simulink model "IEEE9_16b_1"  (R2020a)
settings: Solver=ode15s  StartTime=0.0  StopTime=5  MaxStep=1e-4  RelTol=1e-3
undefined symbols (not defined in the file or in its folder): k
libraries: powerlib_meascontrol x29, powerlib x27, simulink_extras x26, sps_avr x3
(part 1 of 2)
settings Model: Creator=Pankaj  LastModifiedBy=ahmed
settings DataIOCC: ReturnWorkspaceOutputs=off
settings DebuggingCC: UnconnectedInputMsg=none  UnconnectedOutputMsg=none  UnconnectedLineMsg=none  ArithmeticOperatorsInVariantConditions=warning
settings SFSimCC: SimUseLocalCustomCode=off  CustomCodeUndefinedFunction=UseInterfaceOnly
settings RTWCC: RTWUseLocalCustomCode=off
settings CodeAppCC: StateflowObjectComments=on
settings SimscapeCC: SimscapeNormalizeSystem=off

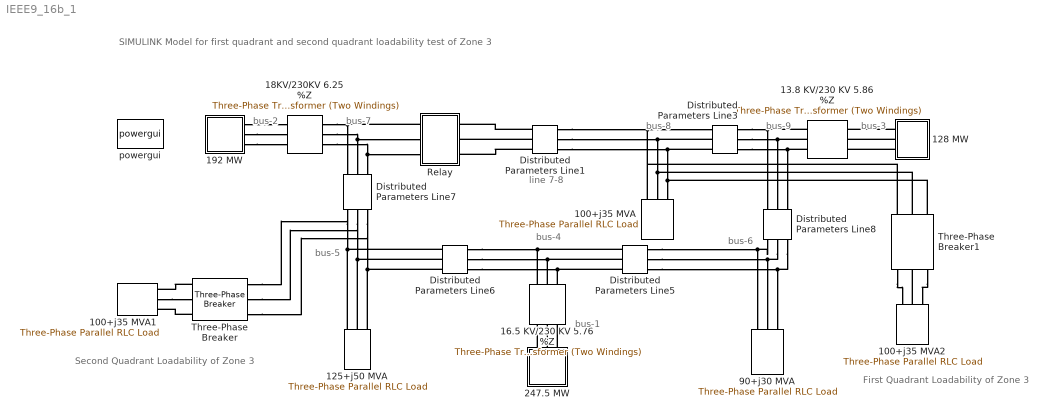
== system IEEE9_16b_1 ==
  note: Second Quadrant Loadability of Zone 3
  note: SIMULINK Model for first quadrant and second quadrant loadability test of Zone 3
  note: bus-2
  note: bus-7
  note: bus-8
  note: bus-9
  note: bus-1
  note: bus-3
  note: bus-4
  note: bus-6
  note: bus-5
  note: line 7-8
  note: First Quadrant Loadability of Zone 3
  100+j35 MVA : powerlib/Elements/Three-Phase Parallel RLC Load  LConnTagsString=A|B|C  Configuration=Y (grounded)  NominalVoltage=(230000)*0.993698  Vabc=[1e3 1e3 1e3]  Vabcp=[1e3 1e3 1e3]  NominalFrequency=60  UnbalancedPower=off  ActivePower=100e6  InductivePower=35e6  CapacitivePower=0  Pabc=[10e3 9e3 11e3]  QLabc=[100 90 110]  QCabc=[100 90 110]  Pabcp=[10e3 9e3 11e3]  QLabcp=[100 90 110]  QCabcp=[100 90 110]  Measurements=None  LoadType=constant PQ
  100+j35 MVA1 : powerlib/Elements/Three-Phase Parallel RLC Load  LConnTagsString=A|B|C  Configuration=Y (grounded)  NominalVoltage=(230000)*0.993698  Vabc=[1e3 1e3 1e3]  Vabcp=[1e3 1e3 1e3]  NominalFrequency=60  UnbalancedPower=off  ActivePower=1.7469e+15  InductivePower=1.0085e+15  CapacitivePower=0  Pabc=[10e3 9e3 11e3]  QLabc=[100 90 110]  QCabc=[100 90 110]  Pabcp=[10e3 9e3 11e3]  QLabcp=[100 90 110]  QCabcp=[100 90 110]  Measurements=None  LoadType=constant PQ
  100+j35 MVA2 : powerlib/Elements/Three-Phase Parallel RLC Load  LConnTagsString=A|B|C  Configuration=Y (grounded)  NominalVoltage=(230000)*0.993698  Vabc=[1e3 1e3 1e3]  Vabcp=[1e3 1e3 1e3]  NominalFrequency=60  UnbalancedPower=off  ActivePower=1.7469e+15  InductivePower=1.0085e+15  CapacitivePower=0  Pabc=[10e3 9e3 11e3]  QLabc=[100 90 110]  QCabc=[100 90 110]  Pabcp=[10e3 9e3 11e3]  QLabcp=[100 90 110]  QCabcp=[100 90 110]  Measurements=None  LoadType=constant PQ
  125+j50 MVA : powerlib/Elements/Three-Phase Parallel RLC Load  LConnTagsString=A|B|C  Configuration=Y (grounded)  NominalVoltage=(223027)*1  Vabc=[1e3 1e3 1e3]  Vabcp=[1e3 1e3 1e3]  NominalFrequency=60  UnbalancedPower=off  ActivePower=125e6  InductivePower=50e6  CapacitivePower=0  Pabc=[10e3 9e3 11e3]  QLabc=[100 90 110]  QCabc=[100 90 110]  Pabcp=[10e3 9e3 11e3]  QLabcp=[100 90 110]  QCabcp=[100 90 110]  Measurements=None  LoadType=constant PQ
  128 MW : Subsystem
  13.8 KV/230 KV 5.86 %Z : powerlib/Elements/Three-Phase Transformer (Two Windings)  Winding1Connection=Yg  Winding2Connection=Yg  CoreType=Three single-phase transformers  SetSaturation=off  Hysteresis=off  DataFile='hysteresis'  SetInitialFlux=off  Measurements=None  UNITS=pu  NominalPower=[ 100e6 , 60 ]  Winding1=[13.8e3 , 1e-6 , 0 ]  Winding2=[ 230e3 , 1e-6, 0.0586 ]  Rm=500  Lm=500  L0=0.5  Saturation=[ 0,0 ; 0.0024,1.2 ; 1.0,1.52 ]  InitialFluxes=[ 0.8 , -0.8 , 0.7 ]  BreakLoop=off  DiscreteSolver=Trapezoidal iterative  DataType=off  TransfoNumber=1
  "16.5 KV/230 KV 5.76 %Z     " : powerlib/Elements/Three-Phase Transformer (Two Windings)  Winding1Connection=Yg  Winding2Connection=Yg  CoreType=Three single-phase transformers  SetSaturation=off  Hysteresis=off  DataFile='hysteresis'  SetInitialFlux=off  Measurements=None  UNITS=pu  NominalPower=[ 100e6 , 60 ]  Winding1=[16.5e3 , 1e-6, 0 ]  Winding2=[ 230e3 ,1e-6, 0.0576 ]  Rm=500  Lm=500  L0=0.5  Saturation=[ 0,0 ; 0.0024,1.2 ; 1.0,1.52 ]  InitialFluxes=[ 0.8 , -0.8 , 0.7 ]  BreakLoop=off  DiscreteSolver=Trapezoidal iterative  DataType=off  TransfoNumber=1
  18KV/230KV 6.25 %Z : powerlib/Elements/Three-Phase Transformer (Two Windings)  Winding1Connection=Yg  Winding2Connection=Yg  CoreType=Three single-phase transformers  SetSaturation=off  Hysteresis=off  DataFile='hysteresis'  SetInitialFlux=off  Measurements=None  UNITS=pu  NominalPower=[ 100e6 , 60 ]  Winding1=[ 18e3 , 1e-6 , 0]  Winding2=[ 230e3 , 1e-6, 0.0625 ]  Rm=500  Lm=500  L0=0.5  Saturation=[ 0,0 ; 0.0024,1.2 ; 1.0,1.52 ]  InitialFluxes=[ 0.8 , -0.8 , 0.7 ]  BreakLoop=off  DiscreteSolver=Trapezoidal iterative  DataType=off  TransfoNumber=1
  192 MW : Subsystem
  247.5 MW : Subsystem
  90+j30 MVA : powerlib/Elements/Three-Phase Parallel RLC Load  LConnTagsString=A|B|C  Configuration=Y (grounded)  NominalVoltage=(226177)*0.999999  Vabc=[1e3 1e3 1e3]  Vabcp=[1e3 1e3 1e3]  NominalFrequency=60  UnbalancedPower=off  ActivePower=90e6  InductivePower=30e6  CapacitivePower=0  Pabc=[10e3 9e3 11e3]  QLabc=[100 90 110]  QCabc=[100 90 110]  Pabcp=[10e3 9e3 11e3]  QLabcp=[100 90 110]  QCabcp=[100 90 110]  Measurements=None  LoadType=constant PQ
  Distributed Parameters Line1 : powerlib/Elements/Distributed Parameters Line  Phases=3  Frequency=60  Resistance=[0.044965 0.11241]  Inductance="[1.01e-3  2.02e-3]"  Capacitance=[12.74e-9 7.751e-9]  Length=100  x1=[-0.0004 1.93656449270455e-06 23508.2160177902 -52538.75935175;-0.00035 1.67378461087068e-06 24494.3184666325 -52086.3350065214;-0.0003 1.4104100413345e-06 25471.7182007562 -51615.4046344802;-0.00025 1.14653435982647e-06 26440.0679546897 -51126.1355549453;-0.0002 8.82251320119748e-07 27399.0236783764 -50618.7016028908;-0.00015 6.17654820719931e-07 28348.2446594139 -50093.2830671837;-0.0001 3.52838871503349e-07 29287.3936441074 -49550.0666265279;-5e-05 8.78975603158065e-08 30216.1369572946 -48989.2452831382]  x2=[-0.0004 4.18624145948892e-06 28259.244689254 -52398.8670670216;-0.00035 3.9633430905482e-06 29241.8663646278 -51856.9185470287;-0.0003 3.73903656467934e-06 30214.0985441207 -51296.5455107989;-0.00025 3.51340157692291e-06 31175.595798269 -50717.9470562037;-0.0002 3.28651829431568e-06 32126.0165116764 -50121.3287565189;-0.00015 3.05846732740762e-06 33065.023004389 -49506.9025873855;-0.0001 2.82932970162139e-06 33992.2816518711 -48874.8868514958;-5e-05 2.59918682846436e-06 34907.4630035407 -48225.5061010312]  x3=[-0.0004 -1.73044531826081e-08 87.9731080176391 -312.019576771818;-0.00035 -1.71851910893741e-08 93.8385916181453 -310.305999768085;-0.0003 -1.70598231795753e-08 99.6707348138731 -308.482172520194;-0.00025 -1.69283939958332e-08 105.467465472116 -306.54874302528;-0.0002 -1.67909502343109e-08 111.226724042071 -304.506398221637;-0.00015 -1.66475407281225e-08 116.946464286594 -302.355863744649;-0.0001 -1.64982164299825e-08 122.624654009211 -300.097903668976;-5e-05 -1.63430303941032e-08 128.259275776149 -297.733320237081]  x4=[-0.0004 3.28235405138543e-08 68.6553647797155 -68.5872480221798;-0.00035 3.17845507984995e-08 69.935937439127 -67.2810236786274;-0.0003 3.07342681835919e-08 71.1916621929746 -65.9508947077285;-0.00025 2.96730658295436e-08 72.4220928882326 -64.5973336979729;-0.0002 2.86013207764978e-08 73.6267923587337 -63.2208215631423;-0.00015 2.75194138103686e-08 74.8053325804924 -61.8218473714436;-0.0001 2.64277293275496e-08 75.9572948237797 -60.400908171746;-5e-05 2.53266551983393e-08 77.0822698018957 -58.9585088169809]  x5=0.000395689524753941  V1=ones(3,3)  V2=ones(3,3)  I1=ones(3,3)  I2=ones(3,3)  nHarmo=1  Measurements=None
  Distributed Parameters Line3 : powerlib/Elements/Distributed Parameters Line  Phases=3  Frequency=60  Resistance=[ 0.062951 0.15737]  Inductance="[ 1.414e-3  3.53e-3]"  Capacitance=[12.74e-9 7.751e-9]  Length=100  x1=[-0.00055 4.84569834764548e-06 0 0;-0.0005 4.62749747611836e-06 0 0;-0.00045 4.40765247677236e-06 27266.5826388019 -52922.198519049;-0.0004 4.18624145948892e-06 28259.244689254 -52398.8670670216;-0.00035 3.9633430905482e-06 29241.8663646278 -51856.9185470287;-0.0003 3.73903656467934e-06 30214.0985441207 -51296.5455107989;-0.00025 3.51340157692291e-06 31175.595798269 -50717.9470562037;-0.0002 3.28651829431568e-06 32126.0165116764 -50121.3287565189;-0.00015 3.05846732740762e-06 33065.023004389 -49506.9025873855;-0.0001 2.82932970162139e-06 33992.2816518711 -48874.8868514958;-5e-05 2.59918682846436e-06 34907.4630035407 -48225.5061010312]  x2=[-0.00055 6.18158400270898e-06 0 0;-0.0005 5.99518973223753e-06 0 0;-0.00045 5.80666539940102e-06 39827.4813836401 -51273.9727441437;-0.0004 5.61607798599722e-06 40786.8453796834 -50514.1819455975;-0.00035 5.42349520682662e-06 41731.7180037748 -49736.4436987352;-0.0003 5.22898548563364e-06 42661.7635471699 -48941.0343302528;-0.00025 5.03261793079605e-06 43576.6515691157 -48128.2364453113;-0.0002 4.83446231077106e-06 44476.0570142543 -47298.338827129;-0.00015 4.63458902930691e-06 45359.6603281138 -46451.6363343782;-0.0001 4.43306910042879e-06 46227.1475706441 -45588.4297964226;-5e-05 4.22997412320786e-06 47078.2105277586 -44709.0259064351]  x3=[-0.00055 -2.65416129090466e-09 0 0;-0.0005 -2.74354657868112e-09 0 0;-0.00045 -2.83195709742188e-09 125.571553781947 -390.764061979304;-0.0004 -2.91936143529064e-09 132.914576268336 -388.327827737904;-0.00035 -3.00572853794231e-09 140.210374838665 -385.753622468377;-0.0003 -3.09102771955659e-09 147.456357330443 -383.042360773598;-0.00025 -3.1752286737404e-09 154.649949280592 -380.195005951937;-0.0002 -3.25830148429566e-09 161.788594840145 -377.212569655006;-0.00015 -3.34021663584833e-09 168.869757682328 -374.096111528218;-0.0001 -3.42094502433513e-09 175.890921903699 -370.846738834307;-5e-05 -3.50045796734401e-09 182.849592918043 -367.465606059919]  x4=[-0.00055 2.18052139273402e-08 0 0;-0.0005 2.13350493540652e-08 0 0;-0.00045 2.0857304539344e-08 48.1436321371247 66.4160212313476;-0.0004 2.03721492236346e-08 46.8832348550945 67.3116503579346;-0.00035 1.98797557803104e-08 45.6061801829603 68.1833639756619;-0.0003 1.93802991544172e-08 44.3129218521663 69.0308523688317;-0.00025 1.88739568005161e-08 43.0039193512395 69.8538144288535;-0.0002 1.83609086196343e-08 41.6796377625354 70.6519577612259;-0.00015 1.78413368953475e-08 40.3405475969968 71.4249987894233;-0.0001 1.73154262290155e-08 38.9871246269832 72.1726628556494;-5e-05 1.67833634741938e-08 37.6198497172315 72.8946843184216]  x5=0.000523077718890797  V1=ones(3,3)  V2=ones(3,3)  I1=ones(3,3)  I2=ones(3,3)  nHarmo=1  Measurements=None
  Distributed Parameters Line5 : powerlib/Elements/Distributed Parameters Line  Phases=3  Frequency=60  Resistance=[ 0.08993 0.224825]  Inductance="[ 1.29e-3  3.22e-3]"  Capacitance=[12.74e-9 7.751e-9]  Length=100  x1=[-0.0005 7.68678845069513e-06 29544.2185806977 -56120.4339666881;-0.00045 7.56630098616658e-06 30596.7580663869 -55553.6046883368;-0.0004 7.44312525092549e-06 31638.4266696252 -54967.0374787648;-0.00035 7.31730500872407e-06 32668.8542905178 -54360.9407425086;-0.0003 7.18888496289525e-06 33687.6748230377 -53735.5298228527;-0.00025 7.05791074046985e-06 34694.5262851008 -53091.0269253187;-0.0002 6.92442887596542e-06 35689.0509471768 -52427.6610387174;-0.00015 6.78848679485286e-06 36670.895459389 -51745.6678537895;-0.0001 6.65013279670626e-06 37639.7109770572 -51045.2896794663;-5e-05 6.50941603804239e-06 38595.1532846412 -50326.7753567781]  x2=[-0.0005 7.53028054430953e-06 29320.5644209634 -55402.7114798878;-0.00045 7.41145500534729e-06 30359.6156210989 -54840.2252139311;-0.0004 7.28999621171217e-06 31387.8801943652 -54258.254477084;-0.00035 7.1659473171352e-06 32404.9928032554 -53657.0060407782;-0.0003 7.03935239559796e-06 33410.5920725029 -53036.6935257204;-0.00025 6.91025642567326e-06 34404.3207174755 -52397.5373259933;-0.0002 6.77870527454453e-06 35385.8256711174 -51739.7645307514;-0.00015 6.64474568170936e-06 36354.7582093921 -51063.6088435367;-0.0001 6.50842524237322e-06 37310.7740751826 -50369.3104992453;-5e-05 6.36979239053909e-06 38253.5336006037 -49657.1161787729]  x3=[-0.0005 1.16182688102649e-08 90.9008008515084 -172.669734952446;-0.00045 1.14361622704147e-08 94.1392240277942 -170.925730953576;-0.0004 1.12499925165645e-08 97.3441999860379 -169.120997856382;-0.00035 1.10598256939413e-08 100.514590013543 -167.256176873939;-0.0003 1.08657293679117e-08 103.649267685827 -165.331930568262;-0.00025 1.06677724999762e-08 106.747119266842 -163.348942614903;-0.0002 1.04660254232673e-08 109.80704410467 -161.307917560037;-0.00015 1.02605598175607e-08 112.827955022586 -159.209580570149;-0.0001 1.00514486838078e-08 115.808778705327 -157.054677174379;-5e-05 9.83876631819869e-09 118.748456080431 -154.843972999644]  x4=[-0.0005 1.31880150263936e-08 63.7477174436907 -184.411908073343;-0.00045 1.30494088536706e-08 67.2122870580504 -183.177608782538;-0.0004 1.29061662881181e-08 70.6529764668576 -181.878227359555;-0.00035 1.27583382231376e-08 74.0685632095486 -180.514225468425;-0.0003 1.26059771813369e-08 77.4578337444175 -179.086087732526;-0.00025 1.24491372958684e-08 80.8195838797816 -177.594321562396;-0.0002 1.22878742911968e-08 84.1526192018252 -176.039456975451;-0.00015 1.21222454632996e-08 87.455755498969 -174.422046407674;-0.0001 1.19523096593109e-08 90.727819182615 -172.742664517341;-5e-05 1.17781272566125e-08 93.9676477041165 -171.001907980839]  x5=0.000499582025297148  V1=ones(3,3)  V2=ones(3,3)  I1=ones(3,3)  I2=ones(3,3)  nHarmo=1  Measurements=None
  Distributed Parameters Line6 : powerlib/Elements/Distributed Parameters Line  Phases=3  Frequency=60  Resistance=[ 0.0529 0.13225]  Inductance="[ 1.192e-3  2.38e-3]"  Capacitance=[12.74e-9 7.751e-9]  Length=100  x1=[-0.00045 -5.95947459759956e-05 0 0;-0.0004 -5.89390235964401e-05 52397.5683409792 -216748.374353491;-0.00035 -5.82623604624459e-05 56473.6196200629 -215722.25524866;-0.0003 -5.75649969892026e-05 60529.6060910015 -214619.491053726;-0.00025 -5.68471809466315e-05 64564.0866811148 -213440.473575556;-0.0002 -5.61091673713546e-05 68575.6279586598 -212185.621713448;-0.00015 -5.53512184760811e-05 72562.804642122 -210855.381310291;-0.0001 -5.45736035564444e-05 76524.2001066113 -209450.224994168;-5e-05 -5.37765988953227e-05 80458.4068871817 -207970.652010426]  x2=[-0.00045 -6.03278555922693e-05 0 0;-0.0004 -5.98632667464564e-05 67525.6481000577 -218721.992470464;-0.00035 -5.93774087670144e-05 71636.2113908087 -217410.381331028;-0.0003 -5.88704542769701e-05 75721.3226767569 -216021.525318331;-0.00025 -5.83425833948398e-05 79779.5305373141 -214555.9178863;-0.0002 -5.77939836706344e-05 83809.393110551 -213014.079758277;-0.00015 -5.72248500192237e-05 87809.478605484 -211396.558742008;-0.0001 -5.66353846510841e-05 91778.3658107837 -209703.929535008;-5e-05 -5.6025797000454e-05 95714.6445997244 -207936.793520373]  x3=[-0.00045 -1.88034187860694e-09 0 0;-0.0004 -1.35212413892515e-09 113.008036792422 -1047.40700837275;-0.00035 -8.23425995975107e-10 132.729903038659 -1045.09091125901;-0.0003 -2.94435293689531e-10 152.404610982357 -1042.40349832082;-0.00025 2.34660020053904e-10 172.025170293465 -1039.3457243832;-0.0002 7.63671960209575e-10 191.584609880685 -1035.91867585868;-0.00015 1.2924125713541e-09 211.075980368268 -1032.12357036127;-0.0001 1.82069399446599e-09 230.492356565089 -1027.96175627389;-5e-05 2.34832853367111e-09 249.826839925139 -1023.43471226927]  x4=[-0.00045 -2.19129648768199e-07 0 0;-0.0004 -2.17997545895897e-07 170.130050868707 -386.485135338421;-0.00035 -2.16787989533558e-07 177.384455284088 -383.209783742097;-0.0003 -2.155014094308e-07 184.575835847143 -379.798279534308;-0.00025 -2.14138262703407e-07 191.701637494601 -376.251834806255;-0.0002 -2.1269903367092e-07 198.759328463067 -372.571709592863;-0.00015 -2.11184233684561e-07 205.746401188547 -368.759211425096;-0.0001 -2.09594400945552e-07 212.66037319737 -364.815694865401;-5e-05 -2.07930100313896e-07 219.498787988203 -360.742561026432]  x5=0.000429504132692574  V1=ones(3,3)  V2=ones(3,3)  I1=ones(3,3)  I2=ones(3,3)  nHarmo=1  Measurements=None
  Distributed Parameters Line7 : powerlib/Elements/Distributed Parameters Line  Phases=3  Frequency=60  Resistance=[ 0.16928 0.4232]  Inductance="[ 2.259e-3  5.64e-3]"  Capacitance=[12.74e-9 7.751e-9]  Length=100  x1=[-0.0007 -2.13875531402635e-06 6576.06110071559 -50761.5133016491;-0.00065 -2.51023483495657e-06 7531.67302268626 -50628.5477731784;-0.0006 -2.88082248140271e-06 8484.60897709492 -50477.5941627577;-0.00055 -3.25038658533858e-06 9434.53039033448 -50308.706103486;-0.0005 -3.61879584239778e-06 10381.09975985 -50121.9436004865;-0.00045 -3.9859193585255e-06 11323.9807740517 -49917.3730095873;-0.0004 -4.35162669648456e-06 12262.8384318048 -49695.0670137453;-0.00035 -4.71578792219914e-06 13197.339161454 -49455.1045972223;-0.0003 -5.07827365091974e-06 14127.1509393399 -49197.5710175221;-0.00025 -5.43895509319298e-06 15051.9434077651 -48922.5577750995;-0.0002 -5.79770410061983e-06 15971.3879923692 -48630.1625808499;-0.00015 -6.15439321138618e-06 16885.1580188692 -48320.4893213936;-0.0001 -6.50889569554939e-06 17792.9288291257 -47993.6480221651;-5e-05 -6.86108560006486e-06 18694.3778964925 -47649.7548083218]  x2=[-0.0007 3.49554589550201e-06 17428.6650067406 -54856.1444386474;-0.00065 3.23828508115508e-06 18459.5267865558 -54517.8978888896;-0.0006 2.97987371953829e-06 19483.8299844009 -54160.2813896054;-0.00055 2.72040362297797e-06 20501.2106702271 -53783.4220002339;-0.0005 2.45996697996393e-06 21511.3073735211 -53387.4536171219;-0.00045 2.19865632239533e-06 22513.761211734 -52972.5169259504;-0.0004 1.93656449270455e-06 23508.2160177902 -52538.75935175;-0.00035 1.67378461087068e-06 24494.3184666325 -52086.3350065214;-0.0003 1.4104100413345e-06 25471.7182007562 -51615.4046344802;-0.00025 1.14653435982647e-06 26440.0679546897 -51126.1355549453;-0.0002 8.82251320119748e-07 27399.0236783764 -50618.7016028908;-0.00015 6.17654820719931e-07 28348.2446594139 -50093.2830671837;-0.0001 3.52838871503349e-07 29287.3936441074 -49550.0666265279;-5e-05 8.78975603158065e-08 30216.1369572946 -48989.2452831382]  x3=[-0.0007 -2.19263741189959e-08 -18.6535496892831 -248.528127503515;-0.00065 -2.17734559243906e-08 -13.9658449001845 -248.835565608354;-0.0006 -2.16128017245723e-08 -9.27317811289293 -249.054593621594;-0.00055 -2.14444685992131e-08 -4.57721660957317 -249.185133723622;-0.0005 -2.1268516356271e-08 0.120371157013008 -249.227139534162;-0.00045 -2.108500751074e-08 4.81791615630025 -249.180596128751;-0.0004 -2.08940072624393e-08 9.51374937291826 -249.045520044038;-0.00035 -2.06955834728475e-08 14.2062023996849 -248.821959271913;-0.0003 -2.04898066409922e-08 18.8936080303834 -248.509993242453;-0.00025 -2.0276749878402e-08 23.5743008521129 -248.109732795705;-0.0002 -2.00564888831302e-08 28.2466178370015 -247.621320142297;-0.00015 -1.98291019128595e-08 32.9088989330721 -247.044928812922;-0.0001 -1.95946697570979e-08 37.5594876540515 -246.380763596672;-5e-05 -1.93532757084738e-08 42.1967316679113 -245.629060468288]  x4=[-0.0007 2.82358103925018e-08 49.0199394768717 -0.498718947797115;-0.00065 2.73756427817605e-08 49.0206313214662 0.425314365616468;-0.0006 2.65057487354913e-08 49.0039063691698 1.34919656686113;-0.00055 2.56264373229066e-08 48.9697705622783 2.27259940498995;-0.0005 2.47380209591643e-08 48.9182360290814 3.19519479937143;-0.00045 2.38408152943683e-08 48.8493210795532 4.11665495625499;-0.0004 2.2935139101419e-08 48.7630501988474 5.03665248523452;-0.00035 2.20213141627554e-08 48.6594540385968 5.95486051556867;-0.0003 2.10996651560268e-08 48.5385694060241 6.87095281231641;-0.00025 2.01705195387369e-08 48.4004392508636 7.78460389224679;-0.0002 1.92342074318991e-08 48.2451126501017 8.69548913948156;-0.00015 1.82910615027468e-08 48.0726447905399 9.60328492082967;-0.0001 1.73414168465375e-08 47.8830969491877 10.5076687007726;-5e-05 1.63856108674959e-08 47.6765364714904 11.4083191560596]  x5=0.000661178039562719  V1=ones(3,3)  V2=ones(3,3)  I1=ones(3,3)  I2=ones(3,3)  nHarmo=1  Measurements=None
  Distributed Parameters Line8 : powerlib/Elements/Distributed Parameters Line  Phases=3  Frequency=60  Resistance=[ 0.20631 0.5157]  Inductance="[ 2.38e-3  6.09e-3]"  Capacitance=[12.74e-9 7.751e-9]  Length=100  x1=[-0.0007 7.97841966236929e-06 25063.9314735538 -57453.9201757617;-0.00065 7.87053977796756e-06 26142.4011326644 -56971.3000027424;-0.0006 7.75986352825922e-06 27211.5825211327 -56468.4381981077;-0.00055 7.6464302359888e-06 28271.0957639024 -55945.5134262624;-0.0005 7.53028020346491e-06 29320.5644209634 -55402.7114798878;-0.00045 7.41145469824105e-06 30359.6156210989 -54840.2252139311;-0.0004 7.28999593845341e-06 31387.8801943652 -54258.254477084;-0.00035 7.16594707782102e-06 32404.9928032554 -53657.0060407782;-0.0003 7.03935219031339e-06 33410.5920725029 -53036.6935257204;-0.00025 6.91025625449124e-06 34404.3207174755 -52397.5373259933;-0.0002 6.77870513752587e-06 35385.8256711174 -51739.7645307514;-0.00015 6.64474557890275e-06 36354.7582093921 -51063.6088435367;-0.0001 6.50842517381518e-06 37310.7740751826 -50369.3104992453;-5e-05 6.36979235625398e-06 38253.5336006037 -49657.1161787729]  x2=[-0.0007 6.72732811486975e-06 34825.3942087243 -54794.4952491998;-0.00065 6.5477182369001e-06 35852.0035042055 -54128.3601017747;-0.0006 6.36578198581861e-06 36865.8747535553 -53442.993405744;-0.00055 6.18158400270898e-06 37866.6477331464 -52738.6386686313;-0.0005 5.99518973223753e-06 38853.9668731044 -52015.546144321;-0.00045 5.80666539940102e-06 39827.4813836401 -51273.9727441437;-0.0004 5.61607798599722e-06 40786.8453796834 -50514.1819455975;-0.00035 5.42349520682662e-06 41731.7180037748 -49736.4436987352;-0.0003 5.22898548563364e-06 42661.7635471699 -48941.0343302528;-0.00025 5.03261793079605e-06 43576.6515691157 -48128.2364453113;-0.0002 4.83446231077106e-06 44476.0570142543 -47298.338827129;-0.00015 4.63458902930691e-06 45359.6603281138 -46451.6363343782;-0.0001 4.43306910042879e-06 46227.1475706441 -45588.4297964226;-5e-05 4.22997412320786e-06 47078.2105277586 -44709.0259064351]  x3=[-0.0007 2.38527071321362e-08 93.2850686371976 -229.508387737295;-0.00065 2.35939388519826e-08 97.5943935722225 -227.709346986195;-0.0006 2.33267877577003e-08 101.869043683918 -225.829402188376;-0.00055 2.30513487668008e-08 106.107500209455 -223.869221279273;-0.0005 2.27677197414463e-08 110.30825724541 -221.829500701828;-0.00045 2.24760014536788e-08 114.469822282812 -219.710965159052;-0.0004 2.21762975496169e-08 118.590716737419 -217.514367356534;-0.00035 2.18687145126307e-08 122.669476475052 -215.240487735015;-0.0003 2.15533616255087e-08 126.704652331799 -212.890134193097;-0.00025 2.12303509316299e-08 130.694810628891 -210.464141800201;-0.0002 2.0899797195156e-08 134.638533682086 -207.963372499873;-0.00015 2.05618178602555e-08 138.534420305361 -205.388714803539;-0.0001 2.02165330093768e-08 142.38108630875 -202.741083474817;-5e-05 1.98640653205832e-08 146.177164990137 -200.021419204513]  x4=[-0.0007 -5.81614874562816e-09 13.9814727332807 -35.1394721246944;-0.00065 -5.82864857092987e-09 14.6413165168806 -34.8697020631362;-0.0006 -5.83907750514813e-09 15.2959583104383 -34.5875429624713;-0.00055 -5.84743184293226e-09 15.9451655228418 -34.2930950724844;-0.0005 -5.85370861602584e-09 16.5887074938599 -33.9864630091089;-0.00045 -5.85790559432126e-09 17.2263555760945 -33.6677557172568;-0.0004 -5.86002128665214e-09 17.8578832162182 -33.3370864321114;-0.00035 -5.86005494132305e-09 18.4830660354676 -32.9945726388951;-0.0003 -5.85800654637665e-09 19.1016819093639 -32.6403360311278;-0.00025 -5.85387682959791e-09 19.7135110466327 -32.2745024673894;-0.0002 -5.84766725825554e-09 20.3183360672949 -31.8972019266032;-0.00015 -5.83938003858067e-09 20.9159420799005 -31.5085684618547;-0.0001 -5.82901811498299e-09 21.5061167578789 -31.1087401527636;-5e-05 -5.81658516900461e-09 22.0886504149771 -30.6978590564241]  x5=0.000687048688231045  V1=ones(3,3)  V2=ones(3,3)  I1=ones(3,3)  I2=ones(3,3)  nHarmo=1  Measurements=None
  Relay : Subsystem
  Three-Phase Breaker : powerlib/Elements/Three-Phase Breaker  InitialState=open  SwitchA=on  SwitchB=on  SwitchC=on  SwitchTimes=1  External=off  BreakerResistance=0.01  SnubberResistance=1e6  SnubberCapacitance=inf  Measurements=None
  Three-Phase Breaker1 : powerlib/Elements/Three-Phase Breaker  InitialState=open  SwitchA=on  SwitchB=on  SwitchC=on  SwitchTimes=1  External=off  BreakerResistance=0.01  SnubberResistance=1e6  SnubberCapacitance=inf  Measurements=None
  powergui : powerlib/powergui  Priority=1  SimulationMode=Discrete  SampleTime=50e-6  frequency=60  Iterations=50  frequencyindice=60  Pbase=100e6  ErrMax=0.0001  UnitsV=kV  UnitsW=MW  buscounter=0  FunctionMessages=off  echomessages=off  EnableUseOfTLC=off  CurrentSourceSwitches=off  DisableSnubberDevices=off  DisableRonSwitches=off  DisableVfSwitches=off  DisplayEquations=off  AutomaticDiscreteSolvers=off  SolverType=Tustin/Backward Euler (TBE)  Interpol=off  ExternalGateDelay=off  methode=off  Ts=100  x0status=blocks  SPID=on  SwTol=0  HookPort=off  NonlinearTolerance=1e-4  nMaxIteration=100  ContinueOnMaxIteration=off  RestoreLinks=warning  ResistiveCurrentMeasurement=off  Frange=[0:2:500]  Ylog=off  Xlog=on  ShowGrid=off  save=off  variable=ZData  structure=0  ZoomFFT=off  StartTime=0.0  cycles=1  DisplayStyle=1  fundamental=60  FreqAxis=off  MaxFrequency=1000  frequencyindicesteady=1  RmsSteady=1  display=off
  connections:
  Distributed Parameters Line1/RConn1 -- Three-Phase Breaker1/RConn1 -- 100+j35 MVA/LConn1 -- Distributed Parameters Line3/LConn1
  Distributed Parameters Line1/RConn2 -- Three-Phase Breaker1/RConn2 -- 100+j35 MVA/LConn2 -- Distributed Parameters Line3/LConn2
  Distributed Parameters Line1/RConn3 -- Distributed Parameters Line3/LConn3 -- Three-Phase Breaker1/RConn3 -- 100+j35 MVA/LConn3
  Distributed Parameters Line5/RConn1 -- Distributed Parameters Line8/LConn1 -- 90+j30 MVA/LConn1
  Distributed Parameters Line5/RConn3 -- Distributed Parameters Line8/LConn3 -- 90+j30 MVA/LConn3
  Distributed Parameters Line6/LConn1 -- 125+j50 MVA/LConn1 -- Three-Phase Breaker/RConn1 -- Distributed Parameters Line7/LConn1
  Distributed Parameters Line6/LConn2 -- 125+j50 MVA/LConn2 -- Three-Phase Breaker/RConn2 -- Distributed Parameters Line7/LConn2
  Distributed Parameters Line6/LConn3 -- 125+j50 MVA/LConn3 -- Three-Phase Breaker/RConn3 -- Distributed Parameters Line7/LConn3
  Distributed Parameters Line3/RConn1 -- 13.8 KV/230 KV 5.86 %Z/RConn1 -- Distributed Parameters Line8/RConn1
  Distributed Parameters Line3/RConn2 -- 13.8 KV/230 KV 5.86 %Z/RConn2 -- Distributed Parameters Line8/RConn2
  Distributed Parameters Line3/RConn3 -- 13.8 KV/230 KV 5.86 %Z/RConn3 -- Distributed Parameters Line8/RConn3
  18KV/230KV 6.25 %Z/RConn1 -- Relay/LConn1 -- Distributed Parameters Line7/RConn1
  18KV/230KV 6.25 %Z/RConn2 -- Distributed Parameters Line7/RConn2 -- Relay/LConn2
  18KV/230KV 6.25 %Z/RConn3 -- Distributed Parameters Line7/RConn3 -- Relay/LConn3
  Distributed Parameters Line5/RConn2 -- Distributed Parameters Line8/LConn2 -- 90+j30 MVA/LConn2
  Distributed Parameters Line6/RConn1 -- "16.5 KV/230 KV 5.76 %Z     "/RConn1 -- Distributed Parameters Line5/LConn1
  Distributed Parameters Line6/RConn2 -- "16.5 KV/230 KV 5.76 %Z     "/RConn2 -- Distributed Parameters Line5/LConn2
  Distributed Parameters Line6/RConn3 -- "16.5 KV/230 KV 5.76 %Z     "/RConn3 -- Distributed Parameters Line5/LConn3
  247.5 MW/RConn1 -- "16.5 KV/230 KV 5.76 %Z     "/LConn1
  247.5 MW/RConn2 -- "16.5 KV/230 KV 5.76 %Z     "/LConn2
  247.5 MW/RConn3 -- "16.5 KV/230 KV 5.76 %Z     "/LConn3
  128 MW/RConn1 -- 13.8 KV/230 KV 5.86 %Z/LConn1
  128 MW/RConn2 -- 13.8 KV/230 KV 5.86 %Z/LConn2
  128 MW/RConn3 -- 13.8 KV/230 KV 5.86 %Z/LConn3
  192 MW/RConn1 -- 18KV/230KV 6.25 %Z/LConn1
  192 MW/RConn2 -- 18KV/230KV 6.25 %Z/LConn2
  192 MW/RConn3 -- 18KV/230KV 6.25 %Z/LConn3
  Distributed Parameters Line1/LConn1 -- Relay/RConn1
  Distributed Parameters Line1/LConn2 -- Relay/RConn2
  Distributed Parameters Line1/LConn3 -- Relay/RConn3
  100+j35 MVA1/LConn2 -- Three-Phase Breaker/LConn2
  Three-Phase Breaker/LConn1 -- 100+j35 MVA1/LConn1
  Three-Phase Breaker/LConn3 -- 100+j35 MVA1/LConn3
  Three-Phase Breaker1/LConn3 -- 100+j35 MVA2/LConn3
  Three-Phase Breaker1/LConn1 -- 100+j35 MVA2/LConn1
  100+j35 MVA2/LConn2 -- Three-Phase Breaker1/LConn2

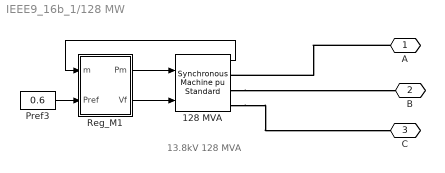
== system IEEE9_16b_1/128 MW ==
  note: 13.8kV 128 MVA
  128 MVA : powerlib/Machines/Synchronous Machine pu Standard  PresetModel=No  MechanicalLoad=Mechanical power Pm  ShowDetailedParameters=on  RotorType=Salient-pole  Units=per unit standard parameters  MeasurementBus=off  NominalParameters="[128e6  13800   60 ]"  Reactances1=[ 31 32 33 34 35 36 37 ]  Reactances2=[ 1.305, 0.296, 0.252, 0.474, 0.243, 0.18 ]  dAxisTimeConstants=Short-circuit  qAxisTimeConstants=Open-circuit  TimeConstants1=[]  TimeConstants2=[]  TimeConstants3=[]  TimeConstants4=[]  TimeConstants5=[ 1.01, 0.053, 0.1 ]  TimeConstants6=[]  TimeConstants7=[]  TimeConstants8=[]  StatorResistance=2.8544e-3  Mechanical="[20 0  32]"  PolePairs=32  InitialConditions=[0 -74.5248 0.603223 0.603223 0.603223 5.08525 -114.915 125.085 1.10339]  SetSaturation=off  Saturation=[0.6404,0.7127,0.8441,0.9214,0.9956,1.082,1.19,1.316,1.457;0.7,0.7698,0.8872,0.9466,0.9969,1.046,1.1,1.151,1.201]  LoadFlowParameters=[1 500000000 0 0 0]  TsPowergui=0  TsBlock=-1  IterativeModel=Trapezoidal non iterative  IterativeDiscreteModel=Trapezoidal non iterative  BusType=PV  Pref=0.6*128e6  Qref=0  Qmin=-Inf  Qmax=Inf  PLF=0  QLF=0
      settings: AttributesFormatString=\n\n
  Pref3 : Constant  Value=0.6
  Reg_M1 : Subsystem
  A : PMIOPort  Side=Right
  B : PMIOPort  Port=2  Side=Right
  C : PMIOPort  Port=3  Side=Right
  wires:
  Reg_M1/1(Pm) -> 128 MVA/1
  Reg_M1/2(Vf) -> 128 MVA/2
  Pref3/1 -> Reg_M1/2(Pref)
  128 MVA/1 -> Reg_M1/1(m)
  connections:
  A/RConn1 -- 128 MVA/RConn1
  128 MVA/RConn2 -- B/RConn1
  128 MVA/RConn3 -- C/RConn1

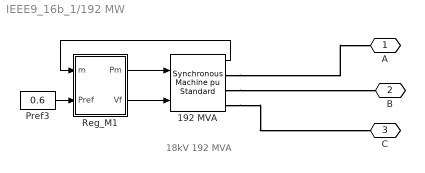
== system IEEE9_16b_1/192 MW ==
  note: 18kV 192 MVA
  192 MVA : powerlib/Machines/Synchronous Machine pu Standard  PresetModel=No  MechanicalLoad=Mechanical power Pm  ShowDetailedParameters=on  RotorType=Salient-pole  Units=per unit standard parameters  MeasurementBus=off  NominalParameters="[192e6  18000   60 ]"  Reactances1=[ 31 32 33 34 35 36 37 ]  Reactances2=[ 1.305, 0.296, 0.252, 0.474, 0.243, 0.18 ]  dAxisTimeConstants=Short-circuit  qAxisTimeConstants=Open-circuit  TimeConstants1=[]  TimeConstants2=[]  TimeConstants3=[]  TimeConstants4=[]  TimeConstants5=[ 1.01, 0.053, 0.1 ]  TimeConstants6=[]  TimeConstants7=[]  TimeConstants8=[]  StatorResistance=2.8544e-3  Mechanical="[20 0  32]"  PolePairs=32  InitialConditions=[0 -73.0594 0.600015 0.600015 0.600015 0.71576 -119.284 120.716 1.18255]  SetSaturation=off  Saturation=[0.6404,0.7127,0.8441,0.9214,0.9956,1.082,1.19,1.316,1.457;0.7,0.7698,0.8872,0.9466,0.9969,1.046,1.1,1.151,1.201]  LoadFlowParameters=[1 500000000 0 0 0]  TsPowergui=0  TsBlock=-1  IterativeModel=Trapezoidal non iterative  IterativeDiscreteModel=Trapezoidal non iterative  BusType=PV  Pref=0.6*192e6  Qref=0  Qmin=-Inf  Qmax=Inf  PLF=0  QLF=0
      settings: AttributesFormatString=\n\n
  Pref3 : Constant  Value=0.6
  Reg_M1 : Subsystem
  A : PMIOPort  Side=Right
  B : PMIOPort  Port=2  Side=Right
  C : PMIOPort  Port=3  Side=Right
  wires:
  Reg_M1/1(Pm) -> 192 MVA/1
  192 MVA/1 -> Reg_M1/1(m)
  Reg_M1/2(Vf) -> 192 MVA/2
  Pref3/1 -> Reg_M1/2(Pref)
  connections:
  192 MVA/RConn1 -- A/RConn1
  192 MVA/RConn3 -- C/RConn1
  192 MVA/RConn2 -- B/RConn1

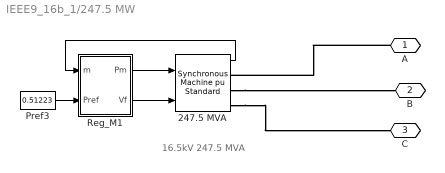
== system IEEE9_16b_1/247.5 MW ==
  note: 16.5kV 247.5 MVA
  247.5 MVA : powerlib/Machines/Synchronous Machine pu Standard  PresetModel=No  MechanicalLoad=Mechanical power Pm  ShowDetailedParameters=on  RotorType=Salient-pole  Units=per unit standard parameters  MeasurementBus=off  NominalParameters="[247.5e6  16500   60 ]"  Reactances1=[ 31 32 33 34 35 36 37 ]  Reactances2=[ 1.305, 0.296, 0.252, 0.474, 0.243, 0.18 ]  dAxisTimeConstants=Short-circuit  qAxisTimeConstants=Open-circuit  TimeConstants1=[]  TimeConstants2=[]  TimeConstants3=[]  TimeConstants4=[]  TimeConstants5=[ 1.01, 0.053, 0.1 ]  TimeConstants6=[]  TimeConstants7=[]  TimeConstants8=[]  StatorResistance=2.8544e-3  Mechanical=[20 0 32]  PolePairs=32  InitialConditions=[0 -76.6925 0.514814 0.514814 0.514814 -5.74321 -125.743 114.257 1.19383]  SetSaturation=off  Saturation=[0.6404,0.7127,0.8441,0.9214,0.9956,1.082,1.19,1.316,1.457;0.7,0.7698,0.8872,0.9466,0.9969,1.046,1.1,1.151,1.201]  LoadFlowParameters=[1 500000000 0 0 0]  TsPowergui=0  TsBlock=-1  IterativeModel=Trapezoidal non iterative  IterativeDiscreteModel=Trapezoidal non iterative  BusType=swing  Pref=5e+008  Qref=0  Qmin=-Inf  Qmax=Inf  PLF=0  QLF=0
      settings: AttributesFormatString=\n\n
  Pref3 : Constant  Value=0.51223
  Reg_M1 : Subsystem
  A : PMIOPort  Side=Right
  B : PMIOPort  Port=2  Side=Right
  C : PMIOPort  Port=3  Side=Right
  wires:
  Reg_M1/1(Pm) -> 247.5 MVA/1
  Reg_M1/2(Vf) -> 247.5 MVA/2
  Pref3/1 -> Reg_M1/2(Pref)
  247.5 MVA/1 -> Reg_M1/1(m)
  connections:
  A/RConn1 -- 247.5 MVA/RConn1
  247.5 MVA/RConn2 -- B/RConn1
  247.5 MVA/RConn3 -- C/RConn1

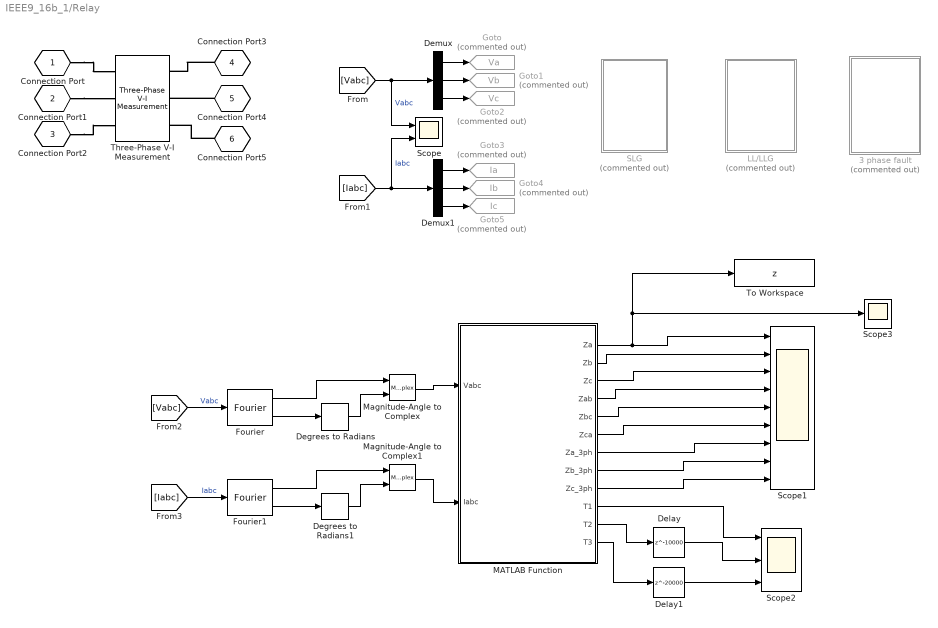
== system IEEE9_16b_1/Relay ==
  3 phase fault : Subsystem  Commented=on
  Degrees to Radians : simulink_extras/Transformations/Degrees to Radians
  Degrees to Radians1 : simulink_extras/Transformations/Degrees to Radians
  Delay : Delay  DelayLength=10000  SampleTime=50e-6
  Delay1 : Delay  DelayLength=20000  SampleTime=50e-6
  Demux : Demux  Outputs=3
  Demux1 : Demux  Outputs=3
  Fourier : powerlib_meascontrol/Measurements/Fourier  Freq=60  n=1  InInit=[0, 0]  Ts=0
  Fourier1 : powerlib_meascontrol/Measurements/Fourier  Freq=60  n=1  InInit=[0, 0]  Ts=0
  Goto : Goto  Commented=on  GotoTag=Va  TagVisibility=global
  Goto1 : Goto  Commented=on  GotoTag=Vb  TagVisibility=global
  Goto2 : Goto  Commented=on  GotoTag=Vc  TagVisibility=global
  Goto3 : Goto  Commented=on  GotoTag=Ia  TagVisibility=global
  Goto4 : Goto  Commented=on  GotoTag=Ib  TagVisibility=global
  Goto5 : Goto  Commented=on  GotoTag=Ic  TagVisibility=global
  LL/LLG : Subsystem  Commented=on
  MATLAB Function : MATLAB Function  TreatAsAtomicUnit=on
  Magnitude-Angle to Complex : MagnitudeAngleToComplex
  Magnitude-Angle to Complex1 : MagnitudeAngleToComplex
  SLG : Subsystem  Commented=on
  Scope : Scope  NumInputPorts=2
  Scope1 : Scope  NumInputPorts=9
  Scope2 : Scope  NumInputPorts=3
  Scope3 : Scope
  Three-Phase V-I Measurement : powerlib/Measurements/Three-Phase V-I Measurement  VoltageMeasurement=phase-to-ground  SetLabelV=on  LabelV=Vabc  Vpu=off  VpuLL=off  CurrentMeasurement=yes  SetLabelI=on  LabelI=Iabc  Ipu=off  Pbase=100e6  Vbase=500e3  OutputType=Complex  PhasorSimulation=off  PSBequivalent=0
  To Workspace : ToWorkspace  VariableName=z  SampleTime=-1
  Connection Port : PMIOPort  Tag=PMCPort  Side=Left
  Connection Port1 : PMIOPort  Tag=PMCPort  Port=2  Side=Left
  Connection Port2 : PMIOPort  Tag=PMCPort  Port=3  Side=Left
  Connection Port3 : PMIOPort  Tag=PMCPort  Port=4  Side=Right
  Connection Port4 : PMIOPort  Tag=PMCPort  Port=5  Side=Right
  Connection Port5 : PMIOPort  Tag=PMCPort  Port=6  Side=Right
  wires:
  Demux1/3 -> Goto5/1
  Demux1/1 -> Goto3/1
  Demux/3 -> Goto2/1
  Demux/1 -> Goto/1
  Demux/2 -> Goto1/1
  [Iabc] -> Scope/2, Demux1/1  "Iabc"
  [Vabc] -> Scope/1, Demux/1  "Vabc"
  Demux1/2 -> Goto4/1
  MATLAB Function/1(Za) -> Scope3/1, To Workspace/1, Scope1/1
  MATLAB Function/2(Zb) -> Scope1/2
  MATLAB Function/3(Zc) -> Scope1/3
  MATLAB Function/4(Zab) -> Scope1/4
  MATLAB Function/5(Zbc) -> Scope1/5
  MATLAB Function/6(Zca) -> Scope1/6
  MATLAB Function/10(T1) -> Scope2/1
  Fourier/2 -> Degrees to Radians/1
  Degrees to Radians/1 -> Magnitude-Angle to Complex/2
  Fourier/1 -> Magnitude-Angle to Complex/1
  Magnitude-Angle to Complex/1 -> MATLAB Function/1(Vabc)
  [Vabc] -> Fourier/1  "Vabc"
  Fourier1/1 -> Magnitude-Angle to Complex1/1
  Degrees to Radians1/1 -> Magnitude-Angle to Complex1/2
  Fourier1/2 -> Degrees to Radians1/1
  [Iabc] -> Fourier1/1  "Iabc"
  Magnitude-Angle to Complex1/1 -> MATLAB Function/2(Iabc)
  MATLAB Function/11(T2) -> Delay/1
  MATLAB Function/12(T3) -> Delay1/1
  Delay/1 -> Scope2/2
  Delay1/1 -> Scope2/3
  MATLAB Function/7(Za_3ph) -> Scope1/7
  MATLAB Function/8(Zb_3ph) -> Scope1/8
  MATLAB Function/9(Zc_3ph) -> Scope1/9
  connections:
  Connection Port/RConn1 -- Three-Phase V-I Measurement/LConn1
  Connection Port1/RConn1 -- Three-Phase V-I Measurement/LConn2
  Connection Port2/RConn1 -- Three-Phase V-I Measurement/LConn3
  Connection Port3/RConn1 -- Three-Phase V-I Measurement/RConn1
  Connection Port4/RConn1 -- Three-Phase V-I Measurement/RConn2
  Connection Port5/RConn1 -- Three-Phase V-I Measurement/RConn3

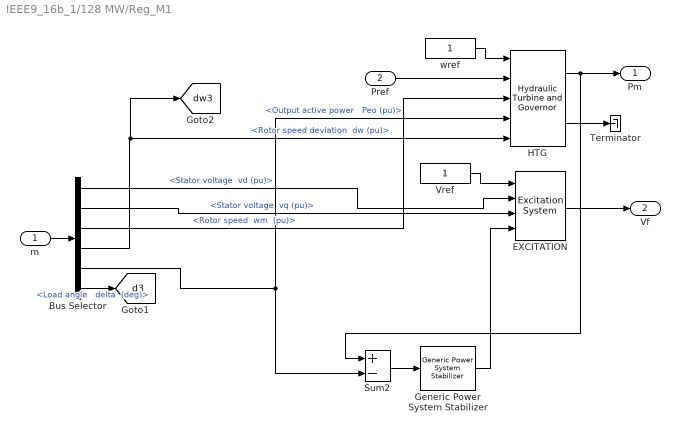
== system IEEE9_16b_1/128 MW/Reg_M1 ==
  m : Inport
  Pref : Inport  Port=2
  Bus Selector : BusSelector  OutputSignals="dq0 components.Stator voltage  vd (pu),dq0 components.Stator voltage  vq (pu),Mechanical.Rotor speed  wm  (pu),Mechanical.Rotor speed deviation  dw (pu),Output active power   Peo (pu),Load angle   delta  (deg)"
  EXCITATION : sps_avr/Excitation System  tr=20e-3  reg=[ 200, 0.001 ]  exc=[ 1, 0 ]  tgr=[ 0, 0 ]  damp=[ 0.001, 0.1 ]  sat=[ 0, 0 ]  lim="[ 0,  7, 0 ]"  v0=[1 1.1034]
      settings: SourceProductBaseCode=PS
  Generic Power System Stabilizer : powerlib/Machines/Generic Power System Stabilizer  Tsensor=15e-3  K=2.5  Twashout=1  Tleadlag1="[0.06  1]"  Tleadlag2="[0  0]"  VSlimits=[-0.15 0.15]  Vinit=0  Plot_On=off  MagdB_On=on  FreqRange=logspace(-2,2,500)
      settings: SourceProductBaseCode=PS
  HTG : powerlib/Machines/Hydraulic Turbine and Governor  sm="[ 10/3  0.07 ]"  gate="[  0.01  0.97518  -0.1  0.1 ]"  reg="[  0.05  1.163  0.105  0  0.01  ]"  hyd="[  0  2.67  ]"  dref=0  po=0.60104
      settings: SourceProductBaseCode=PS
  Sum2 : Sum  Inputs=+-  InputSameDT=on  SaturateOnIntegerOverflow=on  OutDataTypeStr=Inherit: Same as first input
  Terminator : Terminator
  Vref : Constant
  wref : Constant
  Pm : Outport  InitialOutput=0
  Vf : Outport  Port=2  InitialOutput=0
  tag scope: d3=global, dw3=global
  wires:
  HTG/2 -> Terminator/1
  Vref/1 -> EXCITATION/1
  m/1 -> Bus Selector/1
  Bus Selector/4 -> [dw3], HTG/5  "<Rotor speed deviation  dw (pu)>"
  Bus Selector/5 -> HTG/4, Sum2/2  "<Output active power   Peo (pu)>"
  Bus Selector/3 -> HTG/3  "<Rotor speed  wm  (pu)>"
  Pref/1 -> HTG/2
  wref/1 -> HTG/1
  HTG/1 -> Pm/1, Sum2/1
  Bus Selector/2 -> EXCITATION/3  "<Stator voltage  vq (pu)>"
  EXCITATION/1 -> Vf/1
  Bus Selector/1 -> EXCITATION/2  "<Stator voltage  vd (pu)>"
  Generic Power System Stabilizer/1 -> EXCITATION/4
  Sum2/1 -> Generic Power System Stabilizer/1
  Bus Selector/6 -> [d3]  "<Load angle   delta  (deg)>"

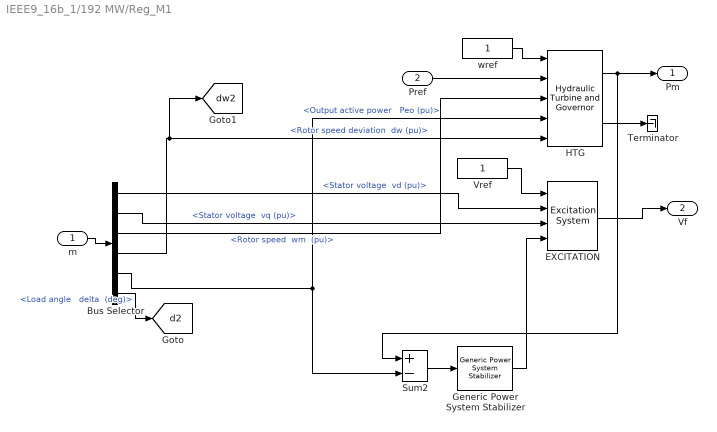
== system IEEE9_16b_1/192 MW/Reg_M1 ==
  m : Inport
  Pref : Inport  Port=2
  Bus Selector : BusSelector  OutputSignals="dq0 components.Stator voltage  vd (pu),dq0 components.Stator voltage  vq (pu),Mechanical.Rotor speed  wm  (pu),Mechanical.Rotor speed deviation  dw (pu),Output active power   Peo (pu),Load angle   delta  (deg)"
  EXCITATION : sps_avr/Excitation System  tr=20e-3  reg=[ 200, 0.001 ]  exc=[ 1, 0 ]  tgr=[ 0, 0 ]  damp=[ 0.001, 0.1 ]  sat=[ 0, 0 ]  lim="[ 0,  7, 0 ]"  v0=[1 1.1826]
      settings: SourceProductBaseCode=PS
  Generic Power System Stabilizer : powerlib/Machines/Generic Power System Stabilizer  Tsensor=15e-3  K=2.5  Twashout=1  Tleadlag1="[0.06  1]"  Tleadlag2="[0  0]"  VSlimits=[-0.15 0.15]  Vinit=0  Plot_On=off  MagdB_On=on  FreqRange=logspace(-2,2,500)
      settings: SourceProductBaseCode=PS
  HTG : powerlib/Machines/Hydraulic Turbine and Governor  sm="[ 10/3  0.07 ]"  gate="[  0.01  0.97518  -0.1  0.1 ]"  reg="[  0.05  1.163  0.105  0  0.01  ]"  hyd="[  0  2.67  ]"  dref=0  po=0.60103
      settings: SourceProductBaseCode=PS
  Sum2 : Sum  Inputs=+-  InputSameDT=on  SaturateOnIntegerOverflow=on  OutDataTypeStr=Inherit: Same as first input
  Terminator : Terminator
  Vref : Constant
  wref : Constant
  Pm : Outport  InitialOutput=0
  Vf : Outport  Port=2  InitialOutput=0
  tag scope: d2=global, dw2=global
  wires:
  HTG/2 -> Terminator/1
  Vref/1 -> EXCITATION/1
  m/1 -> Bus Selector/1
  Bus Selector/4 -> [dw2], HTG/5  "<Rotor speed deviation  dw (pu)>"
  Bus Selector/5 -> HTG/4, Sum2/2  "<Output active power   Peo (pu)>"
  Bus Selector/3 -> HTG/3  "<Rotor speed  wm  (pu)>"
  Pref/1 -> HTG/2
  wref/1 -> HTG/1
  HTG/1 -> Pm/1, Sum2/1
  Bus Selector/2 -> EXCITATION/3  "<Stator voltage  vq (pu)>"
  EXCITATION/1 -> Vf/1
  Bus Selector/1 -> EXCITATION/2  "<Stator voltage  vd (pu)>"
  Generic Power System Stabilizer/1 -> EXCITATION/4
  Sum2/1 -> Generic Power System Stabilizer/1
  Bus Selector/6 -> [d2]  "<Load angle   delta  (deg)>"

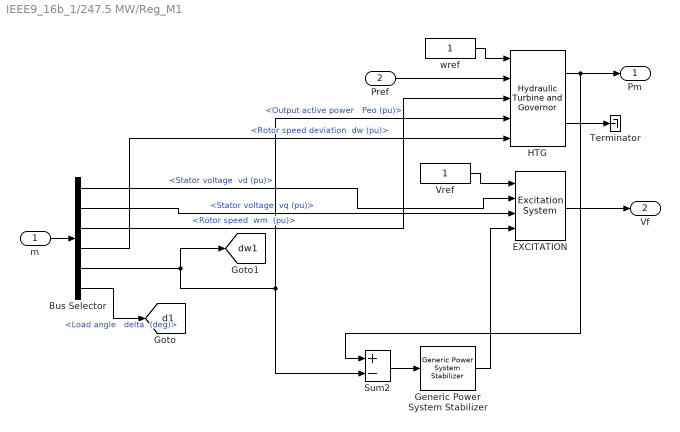
== system IEEE9_16b_1/247.5 MW/Reg_M1 ==
  m : Inport
  Pref : Inport  Port=2
  Bus Selector : BusSelector  OutputSignals="dq0 components.Stator voltage  vd (pu),dq0 components.Stator voltage  vq (pu),Mechanical.Rotor speed  wm  (pu),Mechanical.Rotor speed deviation  dw (pu),Output active power   Peo (pu),Load angle   delta  (deg)"
  EXCITATION : sps_avr/Excitation System  tr=20e-3  reg=[ 200, 0.001 ]  exc=[ 1, 0 ]  tgr=[ 0, 0 ]  damp=[ 0.001, 0.1 ]  sat=[ 0, 0 ]  lim="[ 0,  7, 0 ]"  v0=[1 1.1938]
      settings: SourceProductBaseCode=PS
  Generic Power System Stabilizer : powerlib/Machines/Generic Power System Stabilizer  Tsensor=15e-3  K=2.5  Twashout=1  Tleadlag1="[0.06  1]"  Tleadlag2="[0  0]"  VSlimits=[-0.15 0.15]  Vinit=0  Plot_On=off  MagdB_On=on  FreqRange=logspace(-2,2,500)
      settings: SourceProductBaseCode=PS
  HTG : powerlib/Machines/Hydraulic Turbine and Governor  sm="[ 10/3  0.07 ]"  gate="[  0.01  0.97518  -0.1  0.1 ]"  reg="[  0.05  1.163  0.105  0  0.01  ]"  hyd="[  0  2.67  ]"  dref=0  po=0.51299
      settings: SourceProductBaseCode=PS
  Sum2 : Sum  Inputs=+-  InputSameDT=on  SaturateOnIntegerOverflow=on  OutDataTypeStr=Inherit: Same as first input
  Terminator : Terminator
  Vref : Constant
  wref : Constant
  Pm : Outport  InitialOutput=0
  Vf : Outport  Port=2  InitialOutput=0
  tag scope: d1=global, dw1=global
  wires:
  HTG/2 -> Terminator/1
  Vref/1 -> EXCITATION/1
  m/1 -> Bus Selector/1
  Bus Selector/4 -> HTG/5  "<Rotor speed deviation  dw (pu)>"
  Bus Selector/5 -> [dw1], HTG/4, Sum2/2  "<Output active power   Peo (pu)>"
  Bus Selector/3 -> HTG/3  "<Rotor speed  wm  (pu)>"
  Pref/1 -> HTG/2
  wref/1 -> HTG/1
  HTG/1 -> Pm/1, Sum2/1
  Bus Selector/2 -> EXCITATION/3  "<Stator voltage  vq (pu)>"
  EXCITATION/1 -> Vf/1
  Bus Selector/1 -> EXCITATION/2  "<Stator voltage  vd (pu)>"
  Generic Power System Stabilizer/1 -> EXCITATION/4
  Sum2/1 -> Generic Power System Stabilizer/1
  Bus Selector/6 -> [d1]  "<Load angle   delta  (deg)>"

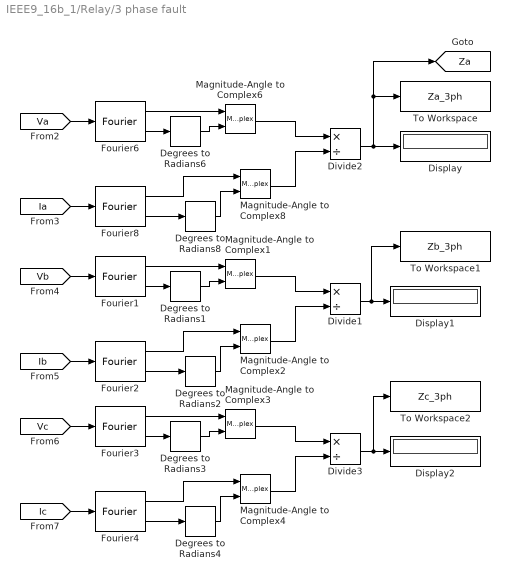
== system IEEE9_16b_1/Relay/3 phase fault ==
  Degrees to Radians{1..4,6,8} (6 alike) : simulink_extras/Transformations/Degrees to Radians
  Display : Display
  Display1 : Display
  Display2 : Display
  Divide1 : Product  Inputs=*/
  Divide2 : Product  Inputs=*/
  Divide3 : Product  Inputs=*/
  Fourier{1..4,6,8} (6 alike) : powerlib_meascontrol/Measurements/Fourier  Freq=60  n=1  InInit=[0, 0]  Ts=0
  Magnitude-Angle to Complex{1..4,6,8} (6 alike) : MagnitudeAngleToComplex
  To Workspace : ToWorkspace  VariableName=Za_3ph  SaveFormat=Timeseries  SampleTime=-1
  To Workspace1 : ToWorkspace  VariableName=Zb_3ph  SaveFormat=Timeseries  SampleTime=-1
  To Workspace2 : ToWorkspace  VariableName=Zc_3ph  SaveFormat=Timeseries  SampleTime=-1
  tag scope: Za=global
  wires:
  Divide1/1 -> To Workspace1/1, Display1/1
  [Ia] -> Fourier8/1
  [Ib] -> Fourier2/1
  Degrees to Radians4/1 -> Magnitude-Angle to Complex4/2
  Magnitude-Angle to Complex3/1 -> Divide3/1
  Fourier4/2 -> Degrees to Radians4/1
  Degrees to Radians8/1 -> Magnitude-Angle to Complex8/2
  Fourier6/2 -> Degrees to Radians6/1
  Magnitude-Angle to Complex6/1 -> Divide2/1
  Magnitude-Angle to Complex8/1 -> Divide2/2
  Degrees to Radians2/1 -> Magnitude-Angle to Complex2/2
  Fourier8/2 -> Degrees to Radians8/1
  [Va] -> Fourier6/1
  Divide3/1 -> To Workspace2/1, Display2/1
  Fourier3/1 -> Magnitude-Angle to Complex3/1
  Degrees to Radians6/1 -> Magnitude-Angle to Complex6/2
  Divide2/1 -> [Za], To Workspace/1, Display/1
  Fourier6/1 -> Magnitude-Angle to Complex6/1
  Fourier8/1 -> Magnitude-Angle to Complex8/1
  Fourier2/2 -> Degrees to Radians2/1
  Fourier3/2 -> Degrees to Radians3/1
  Degrees to Radians1/1 -> Magnitude-Angle to Complex1/2
  [Vc] -> Fourier3/1
  Magnitude-Angle to Complex4/1 -> Divide3/2
  Fourier4/1 -> Magnitude-Angle to Complex4/1
  Fourier1/1 -> Magnitude-Angle to Complex1/1
  Degrees to Radians3/1 -> Magnitude-Angle to Complex3/2
  [Ic] -> Fourier4/1
  Magnitude-Angle to Complex2/1 -> Divide1/2
  Magnitude-Angle to Complex1/1 -> Divide1/1
  Fourier1/2 -> Degrees to Radians1/1
  [Vb] -> Fourier1/1
  Fourier2/1 -> Magnitude-Angle to Complex2/1

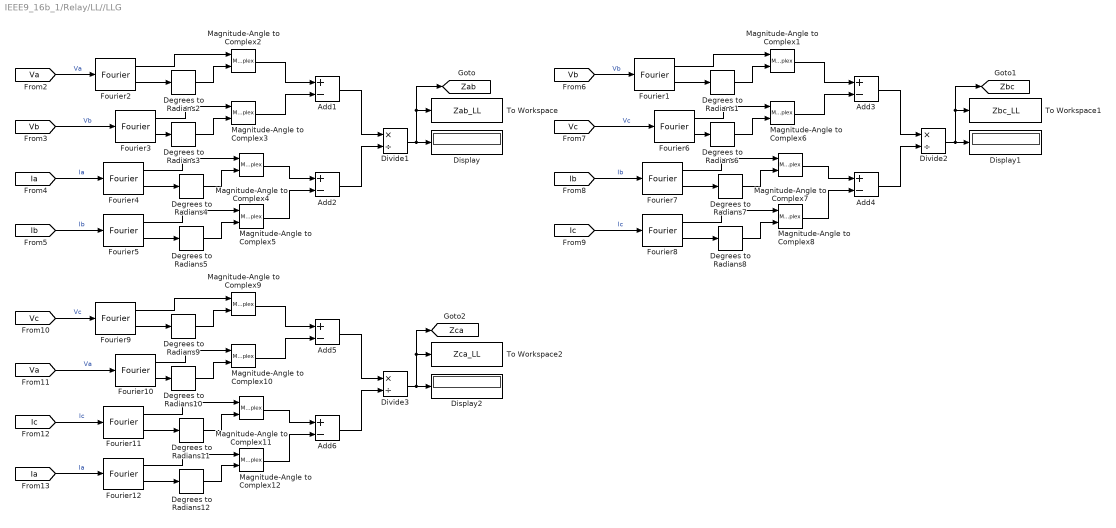
== system IEEE9_16b_1/Relay/LL//LLG ==
  Add{1..6} (6 alike) : Sum  Inputs=+-
  Degrees to Radians{1..12} (12 alike) : simulink_extras/Transformations/Degrees to Radians
  Display : Display
  Display1 : Display
  Display2 : Display
  Divide1 : Product  Inputs=*/
  Divide2 : Product  Inputs=*/
  Divide3 : Product  Inputs=*/
  Fourier{1..12} (12 alike) : powerlib_meascontrol/Measurements/Fourier  Freq=60  n=1  InInit=[0, 0]  Ts=0
  Magnitude-Angle to Complex{1..12} (12 alike) : MagnitudeAngleToComplex
  To Workspace : ToWorkspace  VariableName=Zab_LL  SaveFormat=Timeseries  SampleTime=-1
  To Workspace1 : ToWorkspace  VariableName=Zbc_LL  SaveFormat=Timeseries  SampleTime=-1
  To Workspace2 : ToWorkspace  VariableName=Zca_LL  SaveFormat=Timeseries  SampleTime=-1
  tag scope: Zab=global, Zbc=global, Zca=global
  wires:
  Fourier12/2 -> Degrees to Radians12/1
  [Vc] -> Fourier9/1  "Vc"
  [Vc] -> Fourier6/1  "Vc"
  Magnitude-Angle to Complex11/1 -> Add6/1
  Fourier2/2 -> Degrees to Radians2/1
  Degrees to Radians8/1 -> Magnitude-Angle to Complex8/2
  Fourier10/1 -> Magnitude-Angle to Complex10/1
  Magnitude-Angle to Complex5/1 -> Add2/2
  Add1/1 -> Divide1/1
  Magnitude-Angle to Complex10/1 -> Add5/2
  Fourier3/2 -> Degrees to Radians3/1
  Degrees to Radians7/1 -> Magnitude-Angle to Complex7/2
  Divide2/1 -> Display1/1, [Zbc], To Workspace1/1
  [Va] -> Fourier2/1  "Va"
  Degrees to Radians6/1 -> Magnitude-Angle to Complex6/2
  [Vb] -> Fourier1/1  "Vb"
  Fourier1/2 -> Degrees to Radians1/1
  Fourier3/1 -> Magnitude-Angle to Complex3/1
  [Ib] -> Fourier7/1  "Ib"
  Divide1/1 -> [Zab], To Workspace/1, Display/1
  Degrees to Radians5/1 -> Magnitude-Angle to Complex5/2
  Magnitude-Angle to Complex2/1 -> Add1/1
  Degrees to Radians10/1 -> Magnitude-Angle to Complex10/2
  Fourier8/2 -> Degrees to Radians8/1
  Add3/1 -> Divide2/1
  Fourier8/1 -> Magnitude-Angle to Complex8/1
  [Ic] -> Fourier11/1  "Ic"
  Fourier6/2 -> Degrees to Radians6/1
  Fourier7/2 -> Degrees to Radians7/1
  Fourier5/1 -> Magnitude-Angle to Complex5/1
  [Ic] -> Fourier8/1  "Ic"
  Fourier10/2 -> Degrees to Radians10/1
  Fourier11/2 -> Degrees to Radians11/1
  Degrees to Radians2/1 -> Magnitude-Angle to Complex2/2
  Fourier11/1 -> Magnitude-Angle to Complex11/1
  [Ib] -> Fourier5/1  "Ib"
  Fourier6/1 -> Magnitude-Angle to Complex6/1
  Degrees to Radians3/1 -> Magnitude-Angle to Complex3/2
  Degrees to Radians11/1 -> Magnitude-Angle to Complex11/2
  Fourier7/1 -> Magnitude-Angle to Complex7/1
  Magnitude-Angle to Complex6/1 -> Add3/2
  Fourier2/1 -> Magnitude-Angle to Complex2/1
  Magnitude-Angle to Complex12/1 -> Add6/2
  Magnitude-Angle to Complex8/1 -> Add4/2
  Degrees to Radians9/1 -> Magnitude-Angle to Complex9/2
  [Vb] -> Fourier3/1  "Vb"
  Fourier4/1 -> Magnitude-Angle to Complex4/1
  Add4/1 -> Divide2/2
  Degrees to Radians1/1 -> Magnitude-Angle to Complex1/2
  [Va] -> Fourier10/1  "Va"
  Magnitude-Angle to Complex9/1 -> Add5/1
  Fourier1/1 -> Magnitude-Angle to Complex1/1
  Magnitude-Angle to Complex7/1 -> Add4/1
  [Ia] -> Fourier4/1  "Ia"
  Add2/1 -> Divide1/2
  [Ia] -> Fourier12/1  "Ia"
  Degrees to Radians4/1 -> Magnitude-Angle to Complex4/2
  Fourier4/2 -> Degrees to Radians4/1
  Magnitude-Angle to Complex3/1 -> Add1/2
  Fourier12/1 -> Magnitude-Angle to Complex12/1
  Add6/1 -> Divide3/2
  Degrees to Radians12/1 -> Magnitude-Angle to Complex12/2
  Magnitude-Angle to Complex1/1 -> Add3/1
  Fourier9/2 -> Degrees to Radians9/1
  Add5/1 -> Divide3/1
  Magnitude-Angle to Complex4/1 -> Add2/1
  Fourier5/2 -> Degrees to Radians5/1
  Fourier9/1 -> Magnitude-Angle to Complex9/1
  Divide3/1 -> [Zca], To Workspace2/1, Display2/1
